simulink model "ABS"  (R2020b)
settings: Solver=VariableStepAuto  StartTime=0.0  StopTime=10.0  RelTol=1e-3
PreLoadFcn:
  | initdata
values from neighbouring files (symbols this model uses):
  ctrl = 0    [extraplots.m]
undefined symbols (not defined in the file or in its folder): g, I, Kf, m, mu, PBmax, Rr, slip, TB, v0
settings Model: Creator=abhin  LastModifiedBy=abhin

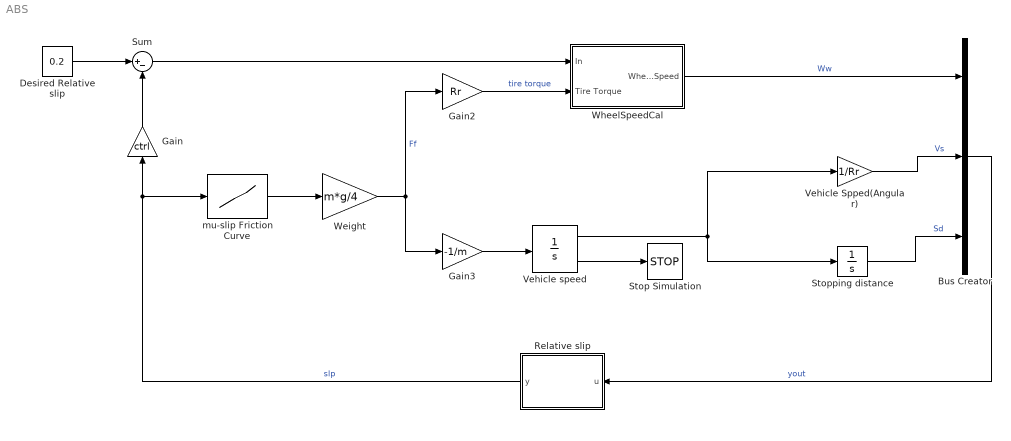
== system ABS ==
  Bus Creator : BusCreator  Inputs=3
  Desired Relative slip : Constant  Value=0.2
  Gain : Gain  Gain=ctrl
  Gain2 : Gain  Gain=Rr
  Gain3 : Gain  Gain=-1/m
  Relative slip : MATLAB Function  TreatAsAtomicUnit=on
  Stop Simulation : Stop
  Stopping distance : Integrator
  Sum : Sum  Inputs=|+-
  Vehicle Spped(Angular) : Gain  Gain=1/Rr
  Vehicle speed : Integrator  InitialCondition=v0  LimitOutput=on  UpperSaturationLimit=1000  LowerSaturationLimit=0  ShowSaturationPort=on
  Weight : Gain  Gain=m*g/4
  WheelSpeedCal : Subsystem
  mu-slip Friction Curve : Lookup_n-D  NumberOfTableDimensions=1  BreakpointsForDimension1=slip  BreakpointsForDimension3=[5, 7]  Table=mu  InternalRulePriority=Speed  RndMeth=Simplest  InputSameDT=on
  wires:
  Desired Relative slip/1 -> Sum/1
  Gain/1 -> Sum/2
  Sum/1 -> WheelSpeedCal/1(In)
  mu-slip Friction Curve/1 -> Weight/1
  Weight/1 -> Gain3/1, Gain2/1  "Ff"
  Gain2/1 -> WheelSpeedCal/2(Tire Torque)  "tire torque"
  Gain3/1 -> Vehicle speed/1
  Vehicle speed/2 -> Stop Simulation/1
  Vehicle speed/1 -> Stopping distance/1, Vehicle Spped(Angular)/1
  WheelSpeedCal/1(WheelSpeed) -> Bus Creator/1  "Ww"
  Vehicle Spped(Angular)/1 -> Bus Creator/2  "Vs"
  Stopping distance/1 -> Bus Creator/3  "Sd"
  Bus Creator/1 -> Relative slip/1(u)  "yout"
  Relative slip/1(y) -> Gain/1, mu-slip Friction Curve/1  "slp"

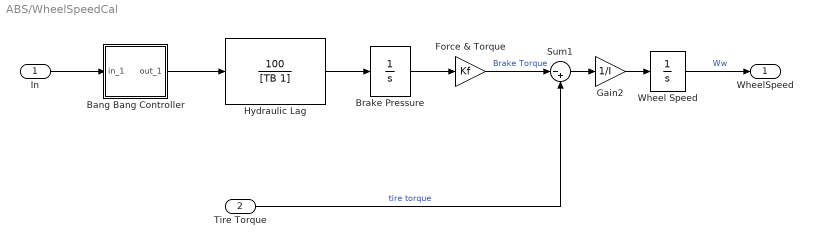
== system ABS/WheelSpeedCal ==
  In : Inport
  Tire Torque : Inport  Port=2
  Bang Bang Controller : Subsystem  mask(Sign){}
      mask help: y = sign(x)
      mask Display: plot(-50,-50,50,50,[-50,50],[0,0],[0,0],[-50,50],[-40,0],[-30,-30],[0,40],[30,30])
  Brake Pressure : Integrator  LimitOutput=on  UpperSaturationLimit=PBmax  LowerSaturationLimit=0
  Force & Torque : Gain  Gain=Kf
  Gain2 : Gain  Gain=1/I
  Hydraulic Lag : TransferFcn  Numerator=[100]  Denominator=[TB 1]
  Sum1 : Sum  Inputs=|-+
  Wheel Speed : Integrator  InitialCondition=v0/Rr  LimitOutput=on  UpperSaturationLimit=1000  LowerSaturationLimit=0
  WheelSpeed : Outport
  wires:
  In/1 -> Bang Bang Controller/1(in_1)
  Tire Torque/1 -> Sum1/2  "tire torque"
  Bang Bang Controller/1(out_1) -> Hydraulic Lag/1
  Force & Torque/1 -> Sum1/1  "Brake Torque"
  Gain2/1 -> Wheel Speed/1
  Sum1/1 -> Gain2/1
  Brake Pressure/1 -> Force & Torque/1
  Hydraulic Lag/1 -> Brake Pressure/1
  Wheel Speed/1 -> WheelSpeed/1  "Ww"

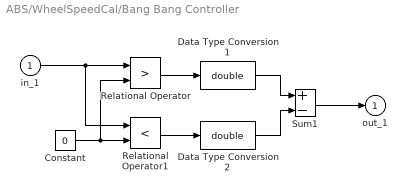
== system ABS/WheelSpeedCal/Bang Bang Controller ==
  in_1 : Inport
  Constant : Constant  Value=0
  Data Type Conversion1 : DataTypeConversion  OutDataTypeStr=double  SaturateOnIntegerOverflow=on  RndMeth=Zero
  Data Type Conversion2 : DataTypeConversion  OutDataTypeStr=double  SaturateOnIntegerOverflow=on  RndMeth=Zero
  Relational Operator : RelationalOperator  Operator=>  OutDataTypeStr=boolean  RndMeth=Nearest  InputSameDT=on
  Relational Operator1 : RelationalOperator  Operator=<  OutDataTypeStr=boolean  RndMeth=Nearest  InputSameDT=on
  Sum1 : Sum  Inputs=+-  InputSameDT=on  SaturateOnIntegerOverflow=on  OutDataTypeStr=Inherit: Same as first input
  out_1 : Outport  InitialOutput=0  VectorParamsAs1DForOutWhenUnconnected=off
  wires:
  in_1/1 -> Relational Operator1/1, Relational Operator/1
  Relational Operator1/1 -> Data Type Conversion2/1
  Constant/1 -> Relational Operator/2, Relational Operator1/2
  Relational Operator/1 -> Data Type Conversion1/1
  Sum1/1 -> out_1/1
  Data Type Conversion1/1 -> Sum1/1
  Data Type Conversion2/1 -> Sum1/2

== matlab function ABS/Relative slip ==
  data: u input; y output
function y = fcn(u)

y = 1.0 - u(1)/(u(2) + (u(2)==0)*eps);
